simulink model "takeoff_13"  (R2024b)
settings: Solver=ode8  StartTime=0.0  StopTime=300  FixedStep=1e-3  MaxStep=1e-3  RelTol=1e-3
values from neighbouring files (symbols this model uses):
  AircraftData =     [AircraftData.mat]
undefined symbols (not defined in the file or in its folder): alpha_dot_0, alpha_g, CD_g_TO, deg, dt_Hold, gamma_c_deg, h_0, k_alpha_Rot, k_CL_max_Rot, magnitude, rad, s
libraries: aerolibconvert2 x6, slpidlib x3, aerolibatmos2 x1, aerolibasang x1
settings Model: Creator=agode  LastModifiedBy=deluc
settings SolverCC: ZeroCrossAlgorithm=Adaptive
settings DebuggingCC: IgnoredZcDiagnostic=none
settings RTWCC: GPUComputeCapability=3.5

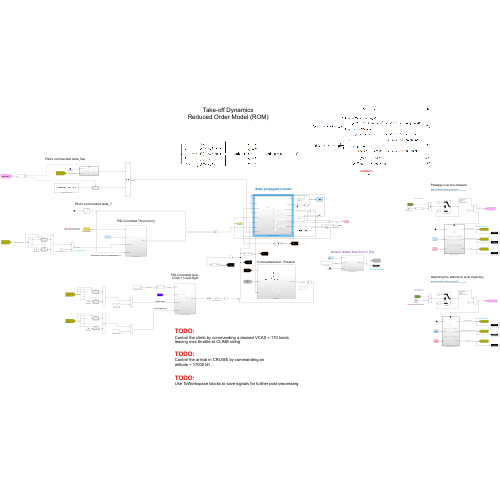
[thumbnail: Simulink's stored preview of the top-level diagram]
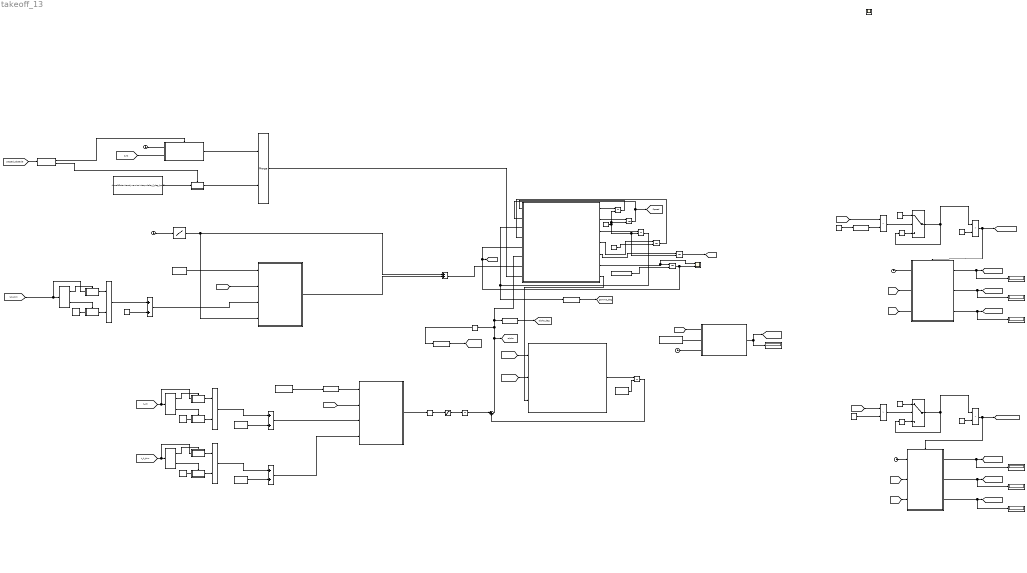
== system takeoff_13 ==
  note: CORRECT:
      | $f_5 = - \dot m_f$
  note: Zero until triggered
  note: Take-off Dynamics
      | Reduced Order Model (ROM)
  note: Detect rotation time from V_Rot
  note: State propagation model
  note: Commanded AoA - Rotation
  note: PID-Controlled AoA - Climb + Level-flight
  note: How to hold the value of a signal?
      | See: https://blogs.mathworks.com/simulink/2014/08/06/how-do-you-hold-the-value-of-a-signal/
  note: Signal may become > X,
      | then < X, then, again > X.
  note: Passage over the obstacle
  note: Zero until triggered
  note: Once this signal
      | becomes = 1,
      | it stays 1
      | (Marcellus Wallace)
  note: Pilot's commanded delta_T
  note: TODO : make this a parameter,
      | taken from performance data
  note: How to hold the value of a signal?
      | See: https://blogs.mathworks.com/simulink/2014/08/06/how-do-you-hold-the-value-of-a-signal/
  note: Zero until triggered
  note: Reaching the altitude to level trajectory
  note: Once this signal
      | becomes = 1,
      | it stays 1
      | (Marcellus Wallace)
  note: Signal may become > X,
      | then < X, then, again > X.
  note: TODO : make this a parameter
  note: PID-Controlled Thrust (trim)
  note: Initial climb
  note: Level trajectory
  note: trim speed: reach a commanded Vc
  note: -1 until triggered
  note: Pilot's commanded delta_flap
  note: TODO:
      | Use ToWorkspace blocks to save signals for further post-processing
  note: TODO:
      | Control the arrival in CRUISE by commanding an altitude = 17000 kft
  note: TODO:
      | Control the climb by commanding a desired VCAS = 170 knots
      | leaving max throttle at CLIMB rating
  1-D Lookup Table : Lookup_n-D  NumberOfTableDimensions=1  BreakpointsForDimension1=[0,2,4,5]  Table=[0, 0.5, 1, 1]  InternalRulePriority=Speed  RndMeth=Simplest
  A/C Reduced Order Dynamics : Subsystem
  Add{,1,3..4} (4 alike) : Sum
  Angle Conversion1 : aerolibconvert2/Angle Conversion  IU=rad  OU=deg
  Angle Conversion2 : aerolibconvert2/Angle Conversion  IU=rad  OU=deg
  Angle Conversion3 : aerolibconvert2/Angle Conversion  IU=deg  OU=rad
  Angular Velocity Conversion3 : aerolibconvert2/Angular Velocity Conversion  IU=rad/s  OU=deg/s
  AoA Control Law in climb : Subsystem
  Clock : Clock
  Clock1 : Clock
  Clock2 : Clock
  Commanded AoA : Subsystem
  Commanded Speed (m/s) : Constant  Value=100
  Commanded gamma (deg) : Constant  Value=gamma_c_deg
  Constant1 : Constant
  Constant2 : Constant  Value=0
  Constant3 : Constant  Value=0
  Constant4 : Constant  Value=alpha_g
  Constant5 : Constant  Value=h_0
  Constant6 : Constant  Value=AircraftData.mass_0
  Constant7 : Constant
  Constant8 : Constant  Value=0
  Derivative : Derivative
  Derivative1 : Derivative
  "Detect S_TO, t_V2, V1" : Subsystem  TreatAsAtomicUnit=on
  "Detect S_TO, t_V2, V2" : Subsystem  TreatAsAtomicUnit=on
  Detect rotation time : Subsystem
  Display{,1..6} (7 alike) : Display
  Flaps at TAKE-OFF position : Constant  Value=AircraftData.Aerodynamics.Interp.delta_f_deg_bp(2)
  Global clock : Clock
  Global clock1 : Clock
  If : If
  If Action Subsystem : Subsystem  TreatAsAtomicUnit=on
  If Action Subsystem1 : Subsystem  TreatAsAtomicUnit=on
  If Action Subsystem2 : Subsystem  TreatAsAtomicUnit=on
  If Action Subsystem3 : Subsystem  TreatAsAtomicUnit=on
  If Action Subsystem4 : Subsystem  TreatAsAtomicUnit=on
  If Action Subsystem5 : Subsystem  TreatAsAtomicUnit=on
  If Action Subsystem6 : Subsystem  TreatAsAtomicUnit=on
  If Action Subsystem7 : Subsystem  TreatAsAtomicUnit=on
  If1 : If
  If2 : If
  If3 : If  IfExpression=u1
  Integrator{,1..6} (7 alike) : Integrator  InitialConditionSource=external
  Integrator7 : Integrator
  Length Conversion : aerolibconvert2/Length Conversion  IU=ft  OU=m
  Memory : Memory
  Memory1 : Memory
  Merge{,1..3} (4 alike) : Merge
  Obstacle height (ft) : Constant  Value=35
  Relational Operator{,1..3} (4 alike) : RelationalOperator  Operator=>  OutDataTypeStr=boolean  RndMeth=Simplest  InputSameDT=off
  Rotation speed : Constant  Value=AircraftData.V_Rot
  Saturation on alpha_dot : Saturate  UpperLimit=12/57.3  LowerLimit=-12/57.3
  Scope : Scope  NumInputPorts=2
  Sum3 : Sum  Inputs=|++
  Switch : Switch  Criteria=u2 > Threshold  SaturateOnIntegerOverflow=off  InputSameDT=off
  Switch1 : Switch  Criteria=u2 > Threshold  SaturateOnIntegerOverflow=off  InputSameDT=off
  Thrust Control Law : Subsystem
  Trim height (m) : Constant  Value=1000
  dummy 0 time : Constant  Value=-11
  level-up decision time (s) : Constant  Value=2
  reaction_time_V2 : Constant  Value=2
  speed-trim decision time (s) : Constant  Value=10
  t_start_climb1 : Constant  Value=1e6
  t_start_climb3 : Constant  Value=1e6
  Angles etc : Scope
  Forces etc : Scope
  tag scope: S_TO=global, S_h_trim=global, Speed=global, alpha=global, alpha_deg=global, alpha_dot_deg_s=global, gamma_deg=global, mass=global, passed_obstacle=global, reached_trim_altitude=global, t_Rot=global, t_V2=global, t_h_trim=global
  wires:
  Commanded AoA/1(AoA_dot (rad/s)) -> Integrator5/1  "alpha_dot (rad/s)"
  Sum3/1 -> Angle Conversion2/1, A/C Reduced Order Dynamics/6(alpha (rad)), Derivative/1, [alpha]
  A/C Reduced Order Dynamics/1(s_dot (m/s)) -> Integrator/1
  A/C Reduced Order Dynamics/2(V_dot (m/s^2)) -> Integrator1/1
  A/C Reduced Order Dynamics/3(gamma_dot (rad/s)) -> Integrator2/1
  A/C Reduced Order Dynamics/4(h_dot (m/s)) -> Integrator3/1
  Integrator1/1 -> A/C Reduced Order Dynamics/2(V (m/s)), [Speed]  "V (m/s)"
  Integrator2/1 -> A/C Reduced Order Dynamics/3(gamma (rad)), Angle Conversion1/1
  Integrator3/1 -> A/C Reduced Order Dynamics/4(h (m))
  Integrator4/1 -> Scope/2, A/C Reduced Order Dynamics/5(mass (kg)), [mass]  "mass (kg)"
  Detect rotation time/1(Rotation time (s)) -> [t_Rot], Display/1
  [Speed] -> Detect rotation time/1(V (m/s))
  Angle Conversion2/1 -> [alpha_deg]  "alpha (deg)"
  Angle Conversion1/1 -> [gamma_deg]  "gamma (deg)"
  Global clock/1 -> Detect rotation time/3(time (s))
  Rotation speed/1 -> Detect rotation time/2(V_Rot (m/s))  "V_Rot (m/s)"
  [t_Rot] -> Commanded AoA/2(t_Rot1)
  [alpha] -> Commanded AoA/1(AoA)
  Integrator5/1 -> Sum3/2
  Commanded gamma (deg)/1 -> Angle Conversion3/1  "gamma_c (deg)"
  Angle Conversion3/1 -> AoA Control Law in climb/1(gamma_c)  "gamma_c"
  [gamma] -> AoA Control Law in climb/2(gamma)
  Angular Velocity Conversion3/1 -> [alpha_dot_deg_s]  "alpha_dot (deg/s)"
  Derivative/1 -> Angular Velocity Conversion3/1
  A/C Reduced Order Dynamics/7(CL) -> Commanded AoA/3(CL)
  A/C Reduced Order Dynamics/6(mass_dot (kg/s)) -> Scope/1, Integrator4/1  "mass_dot (kg/s)"
  A/C Reduced Order Dynamics/5(xE_dot (m/s)) -> Integrator6/1
  Integrator6/1 -> [xE]  "xE (m)"
  [xE] -> "Detect S_TO, t_V2, V2"/3(s (m))
  Relational Operator1/1 -> [passed_obstacle], "Detect S_TO, t_V2, V2"/Trigger
  Constant2/1 -> Relational Operator1/2
  Switch/1 -> Relational Operator1/1, Memory/1
  Relational Operator/1 -> Switch/2
  Memory/1 -> Switch/3
  Constant1/1 -> Switch/1
  [Speed] -> "Detect S_TO, t_V2, V2"/2(V (m/s))
  "Detect S_TO, t_V2, V2"/3(S_ground) -> Display5/1, [S_TO]  "S_TO (m)"
  "Detect S_TO, t_V2, V2"/1(t_LO) -> Display3/1, [t_V2]  "Over-obstacle time (s)"
  "Detect S_TO, t_V2, V2"/2(V_LO) -> Display4/1, [V2_sim]  "Over-obstacle speed sim. (m/s)"
  [h] -> Relational Operator/1
  Clock2/1 -> "Detect S_TO, t_V2, V2"/1(time (s))
  Obstacle height (ft)/1 -> Length Conversion/1
  Length Conversion/1 -> Relational Operator/2
  Integrator/1 -> A/C Reduced Order Dynamics/1(s (m))
  Constant3/1 -> Integrator/2, Integrator1/2, Integrator6/2, Integrator2/2
  Constant5/1 -> Integrator3/2
  Constant6/1 -> Integrator4/2
  Constant4/1 -> Integrator5/2
  Derivative1/1 -> Saturation on alpha_dot/1
  AoA Control Law in climb/1(Delta_alpha) -> Derivative1/1
  Saturation on alpha_dot/1 -> Integrator7/1
  Integrator7/1 -> Sum3/1
  Clock/1 -> 1-D Lookup Table/1
  1-D Lookup Table/1 -> Thrust Control Law/4(Pilot's delta_T), Add/1
  Add/1 -> A/C Reduced Order Dynamics/7(delta_T)
  Thrust Control Law/1(Delta delta_T) -> Add/2
  [Speed] -> Thrust Control Law/2(V)
  Commanded Speed (m/s)/1 -> Thrust Control Law/1(V_c)  "V_c (m/s)"
  reaction_time_V2/1 -> Add1/2
  [t_V2] -> If Action Subsystem/1(In1), If/1
  t_start_climb1/1 -> If Action Subsystem1/1(In1)
  If/1 -> If Action Subsystem/Action
  If/2 -> If Action Subsystem1/Action
  If Action Subsystem/1(Out1) -> Merge/1
  If Action Subsystem1/1(Out1) -> Merge/2
  Merge/1 -> Add1/1
  Add1/1 -> AoA Control Law in climb/3(t_start_climb)
  Constant8/1 -> Relational Operator3/2
  Relational Operator2/1 -> Switch1/2
  [Speed] -> "Detect S_TO, t_V2, V1"/2(V (m/s))
  Memory1/1 -> Switch1/3
  Switch1/1 -> Relational Operator3/1, Memory1/1
  [h] -> Relational Operator2/1
  "Detect S_TO, t_V2, V1"/1(t_h_trim) -> Display1/1, [t_h_trim]  "Level-trajectory time (s)"
  Trim height (m)/1 -> Relational Operator2/2
  Clock1/1 -> "Detect S_TO, t_V2, V1"/1(time (s))
  "Detect S_TO, t_V2, V1"/3(S_h_trim) -> Display6/1, [S_h_trim]  "S_h_trim (m)"
  [xE] -> "Detect S_TO, t_V2, V1"/3(s (m))
  Constant7/1 -> Switch1/1
  "Detect S_TO, t_V2, V1"/2(V_h_trim) -> Display2/1, [V_sim_h_trim]  "Speed at level-trajectory time sim. (m/s)"
  Relational Operator3/1 -> [reached_trim_altitude], "Detect S_TO, t_V2, V1"/Trigger
  If Action Subsystem2/1(Out1) -> Merge1/1
  If Action Subsystem3/1(Out1) -> Merge1/2
  dummy 0 time/1 -> If Action Subsystem3/1(In1)
  If1/1 -> If Action Subsystem2/Action
  If1/2 -> If Action Subsystem3/Action
  [t_h_trim] -> If Action Subsystem4/1(In1), If2/1
  If2/1 -> If Action Subsystem4/Action
  If2/2 -> If Action Subsystem5/Action
  Merge2/1 -> Add3/1
  If Action Subsystem5/1(Out1) -> Merge2/2
  If Action Subsystem4/1(Out1) -> Merge2/1
  level-up decision time (s)/1 -> Add3/2
  t_start_climb3/1 -> If Action Subsystem5/1(In1)
  Add3/1 -> AoA Control Law in climb/4(t_start_level)
  [t_h_trim] -> If Action Subsystem2/1(In1), If1/1  "Level-trajectory trim time (s)"
  speed-trim decision time (s)/1 -> Add4/2
  Merge1/1 -> Add4/1
  Add4/1 -> Thrust Control Law/3(t_start_speed_trim)  "Speed-trim time (s)"
  [passed_obstacle] -> If3/1
  Flaps at TAKE-OFF position/1 -> If Action Subsystem7/1(In1)
  If3/2 -> If Action Subsystem7/Action
  If Action Subsystem7/1(Out1) -> Merge3/2
  Merge3/1 -> A/C Reduced Order Dynamics/8(delta_f (deg))  "delta_f (deg)"
  If3/1 -> If Action Subsystem6/Action
  If Action Subsystem6/1(Out1) -> Merge3/1
  Global clock1/1 -> If Action Subsystem6/1(clock time (s))
  [t_V2] -> If Action Subsystem6/2(t_V2 (s))  "Level-trajectory trim time (s)"

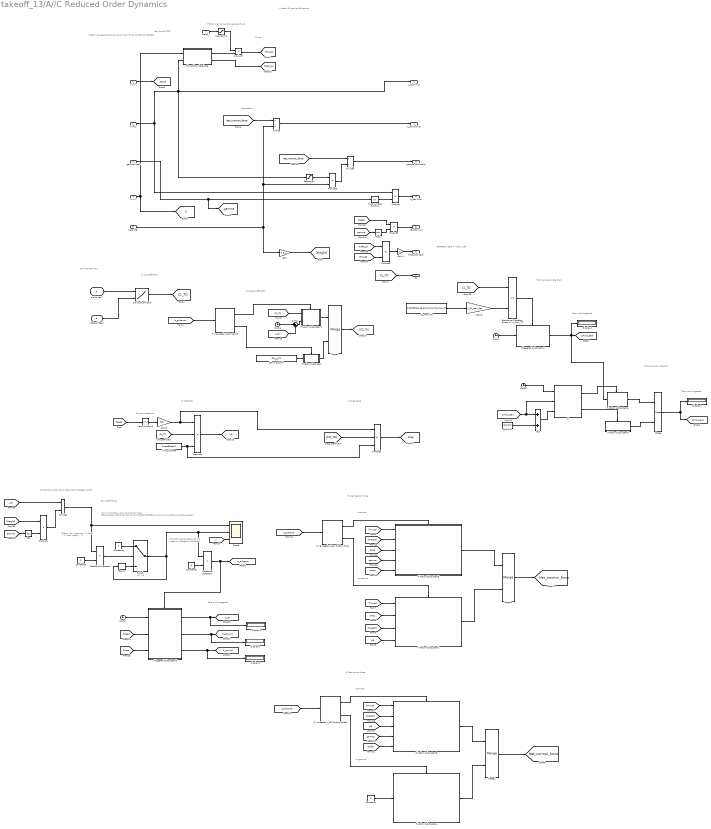
== system takeoff_13/A//C Reduced Order Dynamics ==
  note: TODO: manage the thrust rating, from TO to CLIMB and CRUISE
  note: TODO: plan to handle reverse thrust
  note: on-ground
  note: Commanded
      | AoA
  note: System Dynamics Equations
  note: 3a) Lift-off time
  note: Zero until triggered
  note: 1) Lift coefficient
  note: 3) Lift force
  note: Dinamic pressure
  note: 2) Drag coefficient
  note: 4) Drag force
  note: Max thrust
      | TSFC
  note: 5) Net traction force
  note: Net traction
  note: airborne
  note: 6) Net normal force
  note: on-ground
  note: airborne
  note: Hold AoA grow rate
      | start
  note: Hold AoA grow rate
      | end
  note: Zero until triggered
  note: Zero until triggered
  note: Switching function $S = \frac{L}{W \cos\gamma}$
  note: Once this signal
      | becomes = 1,
      | it stays 1
      | (Marcellus Wallace)
  note: How to hold the value of a signal?
      | See: https://blogs.mathworks.com/simulink/2014/08/06/how-do-you-hold-the-value-of-a-signal/
  note: Signal may become > 1,
      | then < 1, then, again > 1.
  note: Thrust
  note: CORRECT: $f_5 = - \dot m_f$
  s (m) : Inport
  V (m/s) : Inport  Port=2
  gamma (rad) : Inport  Port=3
  h (m) : Inport  Port=4
  mass (kg) : Inport  Port=5
  alpha (rad) : Inport  Port=6
  delta_T : Inport  Port=7  OutDataTypeStr=double
  delta_f (deg) : Inport  Port=8
  2-D Lookup Table : Lookup_n-D  BreakpointsForDimension1=AircraftData.Aerodynamics.Interp.AoA_bp  BreakpointsForDimension2=AircraftData.Aerodynamics.Interp.delta_f_deg_bp  Table=transpose(AircraftData.Aerodynamics.Interp.CL_Interp)  InternalRulePriority=Speed  RndMeth=Simplest
      settings: InputPortMap=u0,u1
  Add : Sum
  CD on ground : Constant  Value=CD_g_TO
  CL_max_TO : Constant  Value=AircraftData.Aerodynamics.CL_max_TO
  Clock{,1..3} (4 alike) : Clock
  Constant1 : Constant  Value=0
  Constant3 : Constant
  Constant4 : Constant
  Constant5 : Constant  Value=0
  Cos : Trigonometry  Operator=cos
  Cos1 : Trigonometry  Operator=cos
  Display{1..5} (5 alike) : Display
  Divide : Product  Inputs=*/
  Divide1 : Product  Inputs=*/
  Divide2 : Product  Inputs=*/
  Gain : Gain  Gain=9.81
  Gain1 : Gain  Gain=-1
  Gain3 : Gain  Gain=k_CL_max_Rot
  Gain5 : Gain  Gain=0.5
  If : If  NumInputs=3  IfExpression=u2 > 0 & u1 > u3
  If Action Subsystem : Subsystem  TreatAsAtomicUnit=on
  If Action Subsystem1 : Subsystem  TreatAsAtomicUnit=on
  If Action Subsystem2 : Subsystem  TreatAsAtomicUnit=on
  If Action Subsystem3 : Subsystem  TreatAsAtomicUnit=on
  If Action Subsystem4 : Subsystem  TreatAsAtomicUnit=on
  If Action Subsystem5 : Subsystem  TreatAsAtomicUnit=on
  If Action Subsystem6 : Subsystem  TreatAsAtomicUnit=on
  If Action Subsystem7 : Subsystem  TreatAsAtomicUnit=on
  If V exceeds V_LO: CD_TO : If  IfExpression=u1
  If V exceeds V_LO: Friction force : If  IfExpression=u1
  If V exceeds V_LO: Friction force1 : If  IfExpression=u1
  Math Function1 : Math  Operator=square
  Memory : Memory
  Merge{,1..3} (4 alike) : Merge
  Product{,3..7} (6 alike) : Product
  Product1 : Product  Inputs=3
  Product2 : Product  Inputs=3
  Relational Operator : RelationalOperator  Operator=>  OutDataTypeStr=boolean  RndMeth=Simplest  InputSameDT=off
  Relational Operator. Event: CL exceed k*CL_max_TO : RelationalOperator  OutDataTypeStr=boolean  RndMeth=Simplest  InputSameDT=off
  Relational Operator1 : RelationalOperator  Operator=>  OutDataTypeStr=boolean  RndMeth=Simplest  InputSameDT=off
  Saturation : Saturate  UpperLimit=1e8  LowerLimit=1e-9
  Saturation1 : Saturate  UpperLimit=1  LowerLimit=0
  Scope : Scope  NumInputPorts=3
  Sum2 : Sum  Inputs=|+-
  Switch : Switch  Criteria=u2 > Threshold  SaturateOnIntegerOverflow=off  InputSameDT=off
  Thrust from database : Subsystem
  Triggered Subsystem1 : Subsystem  TreatAsAtomicUnit=on
  Triggered Subsystem2 : Subsystem  TreatAsAtomicUnit=on
  Trigonometric Function : Trigonometry
  Wing Surface : Constant  Value=AircraftData.S
  dt_Hold1 : Constant  Value=dt_Hold
  s_dot (m/s) : Outport
  V_dot (m/s^2) : Outport  Port=2
  gamma_dot (rad/s) : Outport  Port=3
  h_dot (m/s) : Outport  Port=4
  xE_dot (m/s) : Outport  Port=5
  mass_dot (kg/s) : Outport  Port=6
  CL : Outport  Port=7
  tag scope: CL_TO=global, Drag=global, Lift=global, Net_normal_force=global, Net_traction_force=global, S_ground=global, Space=global, gamma=global, h=global, is_airborne=global, t_Hold_end=global, t_Hold_start=global, t_LO=global
  wires:
  V (m/s)/1 -> Product/1, Saturation/1, Thrust from database/2(Speed (m/s)), s_dot (m/s)/1  "V (m/s)"
  s (m)/1 -> [Space]
  mass (kg)/1 -> Gain/1, Divide/2, Product3/2  "mass (kg)"
  gamma (rad)/1 -> Trigonometric Function/1, [gamma]  "gamma (rad)"
  Trigonometric Function/1 -> Product/2
  Product/1 -> h_dot (m/s)/1
  Triggered Subsystem2/2(V_LO) -> Display4/1, [V_LO_sim]  "Lift-off speed sim. (m/s)"
  Clock2/1 -> Triggered Subsystem2/1(time (s))
  Triggered Subsystem2/1(t_LO) -> [t_LO], Display3/1  "Lift-off time (s)"
  [Speed] -> Triggered Subsystem2/2(V (m/s))
  h (m)/1 -> [h], Thrust from database/1(Altitude (m))  "h (m)"
  [Net_traction_force] -> Divide/1  "Net traction (N)"
  Divide/1 -> V_dot (m/s^2)/1
  2-D Lookup Table/1 -> [CL_TO]  "CL"
  alpha (rad)/1 -> 2-D Lookup Table/1
  Gain5/1 -> Product2/1, Product1/1  "Dynamic pressure (N)"
  Math Function1/1 -> Gain5/1
  Product1/1 -> [Lift]  "Lift (N)"
  [Speed] -> Math Function1/1
  If V exceeds V_LO: CD_TO/1 -> If Action Subsystem1/Action
  [is_airborne] -> If V exceeds V_LO: CD_TO/1  "is_above_V_LO"
  CD on ground/1 -> If Action Subsystem/1(In1)
  Merge2/1 -> [CD_TO]
  If Action Subsystem1/1(CD_TO) -> Merge2/1
  Sum2/1 -> If Action Subsystem1/2(t - t_LO)
  If Action Subsystem/1(Out1) -> Merge2/2
  If V exceeds V_LO: CD_TO/2 -> If Action Subsystem/Action
  [t_LO] -> Sum2/2
  Clock1/1 -> Sum2/1
  [CL_TO] -> If Action Subsystem1/1(CL_TO)
  Product2/1 -> [Drag]  "Drag (N)"
  [CL_TO] -> Product1/2
  Wing Surface/1 -> Product2/3, Product1/3
  [CD_TO] -> Product2/2
  [Drag] -> If Action Subsystem2/2(Drag)
  If Action Subsystem2/1(Net traction force on-ground) -> Merge3/2
  [is_airborne] -> If V exceeds V_LO: Friction force/1  "is_above_V_LO"
  If V exceeds V_LO: Friction force/1 -> If Action Subsystem3/Action
  If Action Subsystem3/1(Net traction force airborne) -> Merge3/1  "Net traction force airborne (N)"
  If V exceeds V_LO: Friction force/2 -> If Action Subsystem2/Action
  Gain/1 -> [Weight]  "Weight (N)"
  Merge3/1 -> [Net_traction_force]  "Net traction force (N)"
  [Lift] -> If Action Subsystem2/4(Lift)
  [Weight] -> If Action Subsystem2/3(Weight)
  [Thrust] -> If Action Subsystem2/1(Thrust)
  [Thrust] -> If Action Subsystem3/1(Thrust)
  [Weight] -> If Action Subsystem3/2(Weight)
  [Drag] -> If Action Subsystem3/3(Drag)
  [Thrust] -> If Action Subsystem5/1(Thrust)
  [Lift] -> If Action Subsystem5/3(Lift)
  [gamma] -> If Action Subsystem5/4(gamma)
  If V exceeds V_LO: Friction force1/2 -> If Action Subsystem4/Action
  If Action Subsystem5/1(Net normal force airborne) -> Merge1/1
  [is_airborne] -> If V exceeds V_LO: Friction force1/1  "is_above_V_LO"
  If Action Subsystem4/1(Net normal force on-ground) -> Merge1/2
  Merge1/1 -> [Net_normal_force]  "Net traction force (N)"
  If V exceeds V_LO: Friction force1/1 -> If Action Subsystem5/Action
  [Weight] -> If Action Subsystem5/2(Weight)
  Constant1/1 -> If Action Subsystem4/1(in1)
  [alpha] -> If Action Subsystem3/5(AoA)
  [gamma] -> If Action Subsystem3/4(gamma)
  [alpha] -> If Action Subsystem5/5(AoA)
  [Net_normal_force] -> Divide1/1  "Net norm. force (N)"
  Product3/1 -> Divide1/2
  Triggered Subsystem1/1(t_Hold_start) -> If Action Subsystem6/1(t_Hold_start), Display2/1, [t_Hold_start]  "Hold time start (s)"
  Clock/1 -> Triggered Subsystem1/1(time (s))
  Relational Operator. Event: CL exceed k*CL_max_TO/1 -> Triggered Subsystem1/Trigger
  CL_max_TO/1 -> Gain3/1  "CL_max"
  Divide1/1 -> gamma_dot (rad/s)/1
  Saturation/1 -> Product3/1
  [CL_TO] -> Relational Operator. Event: CL exceed k*CL_max_TO/1
  Gain3/1 -> Relational Operator. Event: CL exceed k*CL_max_TO/2  "CL_Hold_start"
  [Lift] -> Divide2/1
  [Weight] -> Product4/1
  Cos/1 -> Product4/2
  [gamma] -> Cos/1
  Product4/1 -> Divide2/2
  Divide2/1 -> Relational Operator/1, Scope/1  "Switching func"
  Merge/1 -> [t_Hold_end], Display1/1  "Hold time end (s)"
  Clock3/1 -> If/1
  [t_Hold_start] -> If/2, Add/1
  dt_Hold1/1 -> Add/2
  If/1 -> If Action Subsystem6/Action
  If Action Subsystem6/1(Out1) -> Merge/1
  If Action Subsystem7/1(Zero (s)) -> Merge/2
  If/2 -> If Action Subsystem7/Action
  Add/1 -> If/3
  Constant4/1 -> Switch/1
  Constant3/1 -> Relational Operator/2
  Switch/1 -> Relational Operator1/1, Scope/2, Memory/1
  Relational Operator/1 -> Switch/2
  Memory/1 -> Switch/3
  Constant5/1 -> Relational Operator1/2
  Relational Operator1/1 -> Triggered Subsystem2/Trigger, [is_airborne]
  [h] -> Scope/3
  [Space] -> Triggered Subsystem2/3(s (m))
  Triggered Subsystem2/3(S_ground) -> Display5/1, [S_ground]  "S_ground (m)"
  [CL_TO] -> CL/1
  [Speed] -> Product5/1
  [gamma] -> Cos1/1
  Cos1/1 -> Product5/2
  Product5/1 -> xE_dot (m/s)/1
  [TSFC_SI] -> Product6/1
  [Thrust] -> Product6/2
  Product6/1 -> Gain1/1
  Gain1/1 -> mass_dot (kg/s)/1
  Product7/1 -> [Thrust]  "Thrust (N)"
  Thrust from database/1(Max Thrust (N)) -> Product7/2  "Thrust_max (N)"
  delta_T/1 -> Saturation1/1
  Saturation1/1 -> Product7/1
  Thrust from database/2(TSFC kg/(N*s)) -> [TSFC_SI]
  delta_f (deg)/1 -> 2-D Lookup Table/2

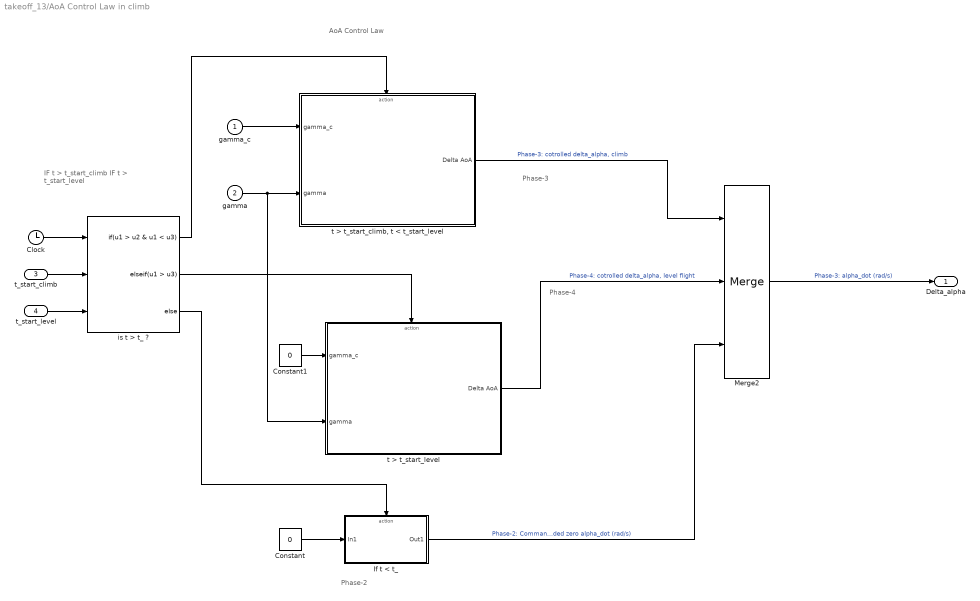
== system takeoff_13/AoA Control Law in climb ==
  note: Phase-3
  note: IF t > t_start_climb
      | IF t > t_start_level
  note: Phase-2
  note: AoA Control Law
  note: Phase-4
  gamma_c : Inport
  gamma : Inport  Port=2
  t_start_climb : Inport  Port=3
  t_start_level : Inport  Port=4
  Clock : Clock
  Constant : Constant  Value=0
  Constant1 : Constant  Value=0
  If t < t_ : Subsystem  TreatAsAtomicUnit=on
  Merge2 : Merge  Inputs=3
  is t > t_ ? : If  NumInputs=3  IfExpression=u1 > u2 & u1 < u3  ElseIfExpressions=u1 > u3
  "t > t_start_climb, t < t_start_level" : Subsystem  TreatAsAtomicUnit=on
  t > t_start_level : Subsystem  TreatAsAtomicUnit=on
  Delta_alpha : Outport
  wires:
  gamma_c/1 -> "t > t_start_climb, t < t_start_level"/1(gamma_c)
  gamma/1 -> t > t_start_level/2(gamma), "t > t_start_climb, t < t_start_level"/2(gamma)
  If t < t_/1(Out1) -> Merge2/3  "Phase-2: Commanded zero alpha_dot (rad/s)"
  t_start_climb/1 -> is t > t_ ?/2
  "t > t_start_climb, t < t_start_level"/1(Delta AoA) -> Merge2/1  "Phase-3: cotrolled delta_alpha, climb"
  is t > t_ ?/1 -> "t > t_start_climb, t < t_start_level"/Action
  is t > t_ ?/3 -> If t < t_/Action
  Constant/1 -> If t < t_/1(In1)
  Merge2/1 -> Delta_alpha/1  "Phase-3: alpha_dot (rad/s)"
  Clock/1 -> is t > t_ ?/1
  t_start_level/1 -> is t > t_ ?/3
  is t > t_ ?/2 -> t > t_start_level/Action
  Constant1/1 -> t > t_start_level/1(gamma_c)
  t > t_start_level/1(Delta AoA) -> Merge2/2  "Phase-4: cotrolled delta_alpha, level flight"

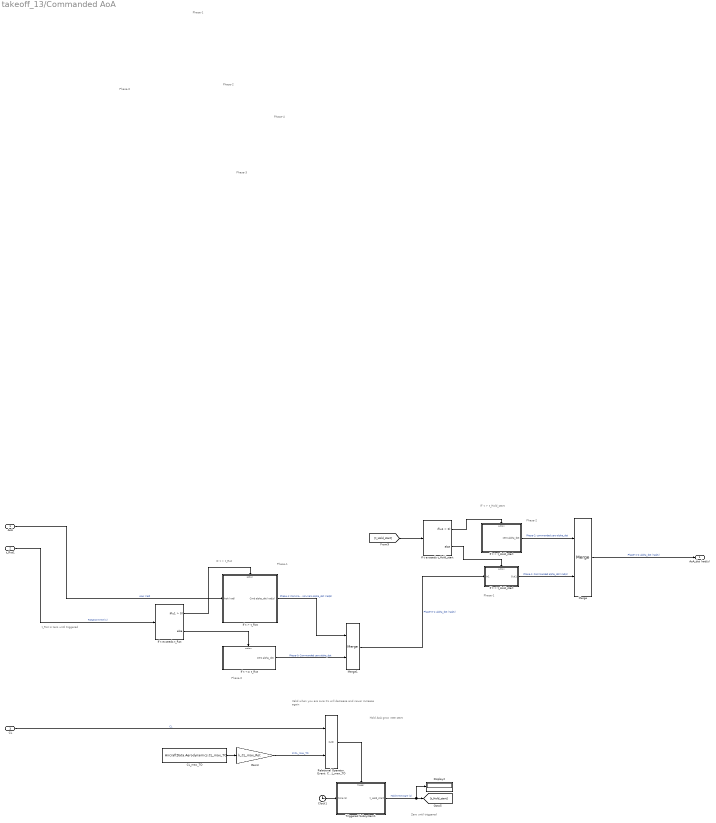
== system takeoff_13/Commanded AoA ==
  note: IF t > t_Rot
  note: t_Rot is zero until triggered
  note: Hold AoA grow rate
      | start
  note: Zero until triggered
  note: IF t > t_Hold_start
  note: Valid when you are sure CL will decrease and never increase again
  note: Phase-0
  note: Phase-1
  note: Phase-2
  note: Phase-3
  note: Phase-4
  note: Phase-0
  note: Phase-1
  note: Phase-1
  note: Phase-2
  AoA : Inport
  t_Rot1 : Inport  Port=2
  CL : Inport  Port=3
  CL_max_TO : Constant  Value=AircraftData.Aerodynamics.CL_max_TO
  Clock1 : Clock
  Display2 : Display
  Gain3 : Gain  Gain=k_CL_max_Rot
  If t < t_Hold_start : Subsystem  TreatAsAtomicUnit=on
  If t <= t_Rot : Subsystem  TreatAsAtomicUnit=on
  If t > t_Hold_start : Subsystem  TreatAsAtomicUnit=on
  If t > t_Rot : Subsystem  TreatAsAtomicUnit=on
  If t exceeds t_Hold_start : If
  If t exceeds t_Rot : If
  Merge : Merge
  Merge1 : Merge
  Relational Operator. Event: CL exceed k*CL_max_TO : RelationalOperator  OutDataTypeStr=boolean  RndMeth=Simplest  InputSameDT=off
  Triggered Subsystem1 : Subsystem  TreatAsAtomicUnit=on
  AoA_dot (rad/s) : Outport
  wires:
  If t > t_Rot/1(Cmd alpha_dot (rad/s)) -> Merge1/1  "Phase-1: Commanded non-zero alpha_dot (rad/s)"
  t_Rot1/1 -> If t exceeds t_Rot/1  "Rotation time (s)"
  If t exceeds t_Rot/2 -> If t <= t_Rot/Action
  If t <= t_Rot/1(zero alpha_dot) -> Merge1/2  "Phase-0: Commanded zero alpha_dot"
  AoA/1 -> If t > t_Rot/1(AoA (rad))  "AoA (rad)"
  If t exceeds t_Rot/1 -> If t > t_Rot/Action
  Triggered Subsystem1/1(t_Hold_start) -> Display2/1, [t_Hold_start]  "Hold time start (s)"
  Clock1/1 -> Triggered Subsystem1/1(time (s))
  Relational Operator. Event: CL exceed k*CL_max_TO/1 -> Triggered Subsystem1/Trigger
  CL_max_TO/1 -> Gain3/1
  Gain3/1 -> Relational Operator. Event: CL exceed k*CL_max_TO/2  "k*CL_max_TO"
  CL/1 -> Relational Operator. Event: CL exceed k*CL_max_TO/1  "CL"
  If t < t_Hold_start/1(Out1) -> Merge/2  "Phase-1: Commanded alpha_dot (rad/s)"
  If t exceeds t_Hold_start/1 -> If t > t_Hold_start/Action
  Merge1/1 -> If t < t_Hold_start/1(In1)  "Phase-0-1: alpha_dot (rad/s)"
  If t exceeds t_Hold_start/2 -> If t < t_Hold_start/Action
  If t > t_Hold_start/1(zero alpha_dot) -> Merge/1  "Phase-2: commanded zero alpha_dot"
  [t_Hold_start] -> If t exceeds t_Hold_start/1
  Merge/1 -> AoA_dot (rad/s)/1  "Phase-1-2: alpha_dot (rad/s)"

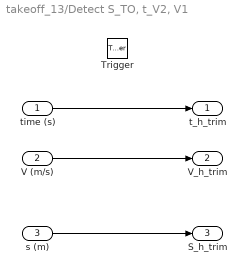
== system takeoff_13/Detect S_TO, t_V2, V1 ==
  time (s) : Inport
  V (m/s) : Inport  Port=2
  s (m) : Inport  Port=3
  Trigger : TriggerPort  VariantControl=(inherit)
  t_h_trim : Outport
  V_h_trim : Outport  Port=2
  S_h_trim : Outport  Port=3
  wires:
  time (s)/1 -> t_h_trim/1
  V (m/s)/1 -> V_h_trim/1
  s (m)/1 -> S_h_trim/1

== system takeoff_13/Detect S_TO, t_V2, V2 ==
  time (s) : Inport
  V (m/s) : Inport  Port=2
  s (m) : Inport  Port=3
  Trigger : TriggerPort  VariantControl=(inherit)
  t_LO : Outport
  V_LO : Outport  Port=2
  S_ground : Outport  Port=3
  wires:
  time (s)/1 -> t_LO/1
  V (m/s)/1 -> V_LO/1
  s (m)/1 -> S_ground/1

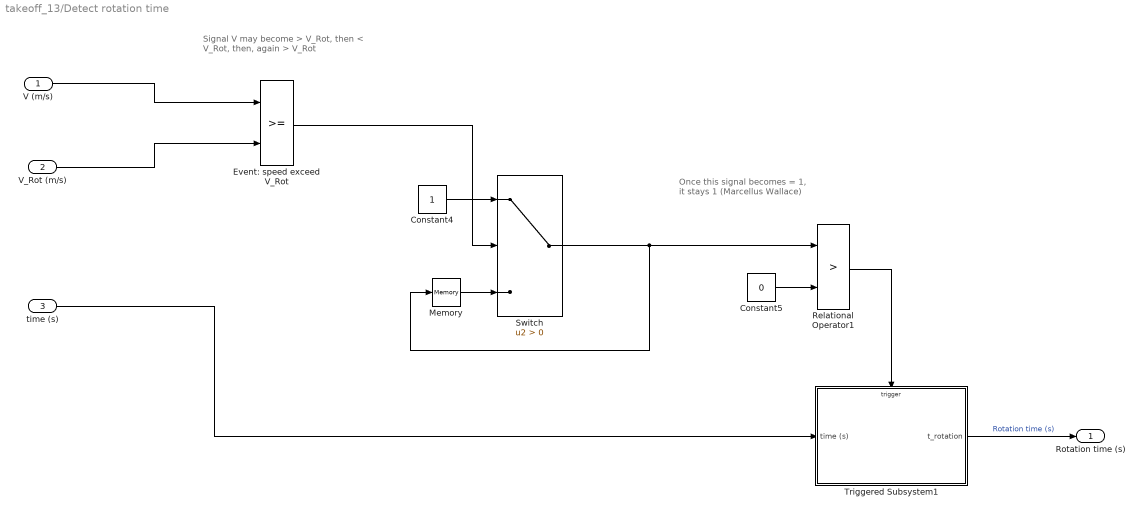
== system takeoff_13/Detect rotation time ==
  note: Signal V may become > V_Rot,
      | then < V_Rot, then, again > V_Rot
  note: Once this signal
      | becomes = 1,
      | it stays 1
      | (Marcellus Wallace)
  V (m/s) : Inport
  V_Rot (m/s) : Inport  Port=2
  time (s) : Inport  Port=3
  Constant4 : Constant
  Constant5 : Constant  Value=0
  Event: speed exceed V_Rot : RelationalOperator  OutDataTypeStr=boolean  RndMeth=Simplest  InputSameDT=off
  Memory : Memory
  Relational Operator1 : RelationalOperator  Operator=>  OutDataTypeStr=boolean  RndMeth=Simplest  InputSameDT=off
  Switch : Switch  Criteria=u2 > Threshold  SaturateOnIntegerOverflow=off  InputSameDT=off
  Triggered Subsystem1 : Subsystem  TreatAsAtomicUnit=on
  Rotation time (s) : Outport
  wires:
  V (m/s)/1 -> Event: speed exceed V_Rot/1
  time (s)/1 -> Triggered Subsystem1/1(time (s))
  Event: speed exceed V_Rot/1 -> Switch/2
  Switch/1 -> Relational Operator1/1, Memory/1
  Memory/1 -> Switch/3
  V_Rot (m/s)/1 -> Event: speed exceed V_Rot/2
  Constant4/1 -> Switch/1
  Constant5/1 -> Relational Operator1/2
  Relational Operator1/1 -> Triggered Subsystem1/Trigger
  Triggered Subsystem1/1(t_rotation) -> Rotation time (s)/1  "Rotation time (s)"

== system takeoff_13/If Action Subsystem ==
  In1 : Inport
  Action Port : ActionPort  ActionPortLabel=if(u1 > 0)
  Out1 : Outport
  wires:
  In1/1 -> Out1/1

== system takeoff_13/If Action Subsystem1 ==
  In1 : Inport
  Action Port : ActionPort  ActionPortLabel=else
  Out1 : Outport
  wires:
  In1/1 -> Out1/1

== system takeoff_13/If Action Subsystem2 ==
  In1 : Inport
  Action Port : ActionPort  ActionPortLabel=if(u1 > 0)
  Out1 : Outport
  wires:
  In1/1 -> Out1/1

== system takeoff_13/If Action Subsystem3 ==
  In1 : Inport
  Action Port : ActionPort  ActionPortLabel=else
  Out1 : Outport
  wires:
  In1/1 -> Out1/1

== system takeoff_13/If Action Subsystem4 ==
  In1 : Inport
  Action Port : ActionPort  ActionPortLabel=if(u1 > 0)
  Out1 : Outport
  wires:
  In1/1 -> Out1/1

== system takeoff_13/If Action Subsystem5 ==
  In1 : Inport
  Action Port : ActionPort  ActionPortLabel=else
  Out1 : Outport
  wires:
  In1/1 -> Out1/1

== system takeoff_13/If Action Subsystem6 ==
  clock time (s) : Inport
  t_V2 (s) : Inport  Port=2
  Action Port : ActionPort  ActionPortLabel=if(u1)
  1-D Lookup Table: delay then ramp down to CLEAN CL(alpha) : Lookup_n-D  NumberOfTableDimensions=1  BreakpointsForDimension1=[0, 5 + 1.5*[0:5,6]]  Table="AircraftData.Aerodynamics.Interp.delta_f_deg_bp(2)*[1,(1 -  [tanh([0:5]),1])]"  InternalRulePriority=Speed  RndMeth=Simplest
  Add : Sum  Inputs=+-
  Scope : Scope
  Out1 : Outport
  wires:
  clock time (s)/1 -> Add/1
  t_V2 (s)/1 -> Add/2
  Add/1 -> 1-D Lookup Table: delay then ramp down to CLEAN CL(alpha)/1
  1-D Lookup Table: delay then ramp down to CLEAN CL(alpha)/1 -> Scope/1, Out1/1

== system takeoff_13/If Action Subsystem7 ==
  In1 : Inport
  Action Port : ActionPort  ActionPortLabel=else
  Out1 : Outport
  wires:
  In1/1 -> Out1/1

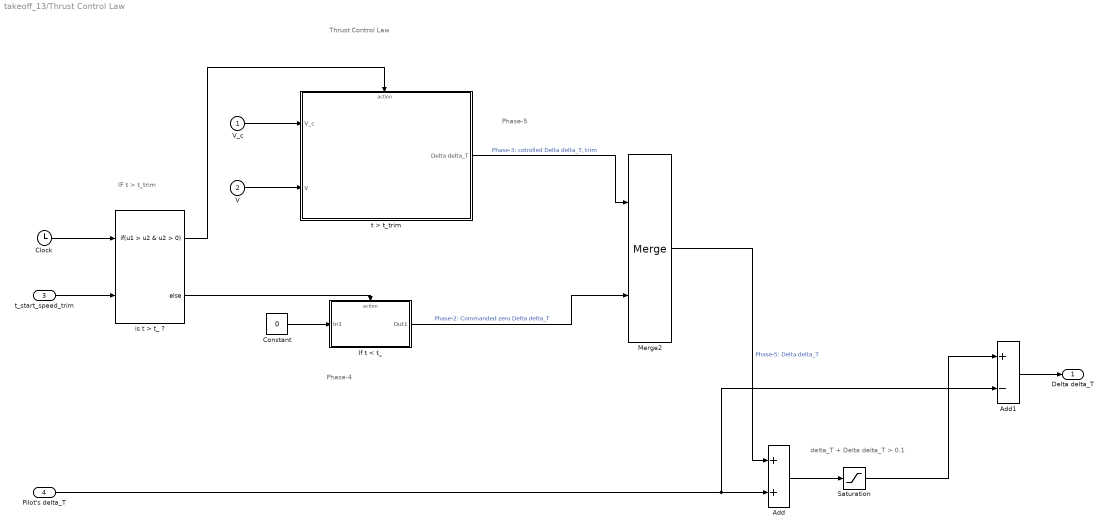
== system takeoff_13/Thrust Control Law ==
  note: delta_T + Delta delta_T > 0.1
  note: Phase-5
  note: IF t > t_trim
  note: Phase-4
  note: Thrust Control Law
  V_c : Inport
  V : Inport  Port=2
  t_start_speed_trim : Inport  Port=3
  Pilot's delta_T : Inport  Port=4
  Add : Sum
  Add1 : Sum  Inputs=+-
  Clock : Clock
  Constant : Constant  Value=0
  If t < t_ : Subsystem  TreatAsAtomicUnit=on
  Merge2 : Merge
  Saturation : Saturate  UpperLimit=1  LowerLimit=0.1
  is t > t_ ? : If  NumInputs=2  IfExpression=u1 > u2 & u2 > 0
  t > t_trim : Subsystem  TreatAsAtomicUnit=on
  Delta delta_T : Outport
  wires:
  V_c/1 -> t > t_trim/1(V_c)
  V/1 -> t > t_trim/2(V)
  If t < t_/1(Out1) -> Merge2/2  "Phase-2: Commanded zero Delta delta_T"
  t_start_speed_trim/1 -> is t > t_ ?/2
  t > t_trim/1(Delta delta_T) -> Merge2/1  "Phase-3: cotrolled Delta delta_T, trim"
  is t > t_ ?/1 -> t > t_trim/Action
  is t > t_ ?/2 -> If t < t_/Action
  Constant/1 -> If t < t_/1(In1)
  Merge2/1 -> Add/1  "Phase-5: Delta delta_T"
  Clock/1 -> is t > t_ ?/1
  Pilot's delta_T/1 -> Add1/2, Add/2
  Add/1 -> Saturation/1
  Saturation/1 -> Add1/1
  Add1/1 -> Delta delta_T/1

== system takeoff_13/A//C Reduced Order Dynamics/If Action Subsystem ==
  In1 : Inport
  Action Port : ActionPort  ActionPortLabel=else
  Out1 : Outport
  wires:
  In1/1 -> Out1/1

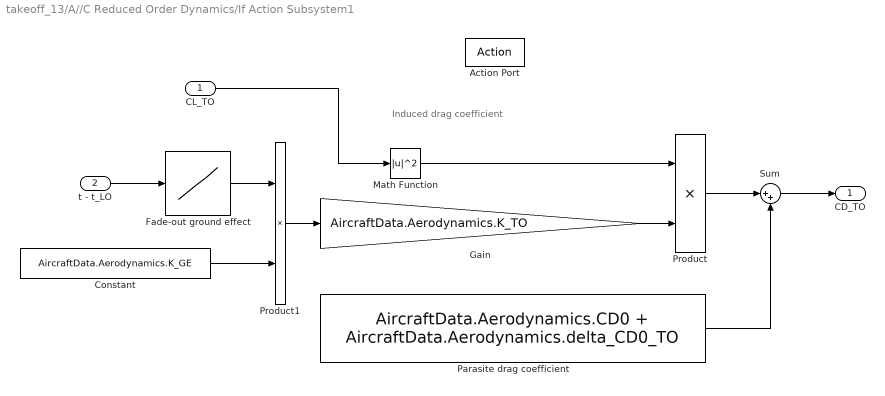
== system takeoff_13/A//C Reduced Order Dynamics/If Action Subsystem1 ==
  note: Induced drag coefficient
  CL_TO : Inport
  t - t_LO : Inport  Port=2
  Action Port : ActionPort  ActionPortLabel=if(u1)
  Constant : Constant  Value=AircraftData.Aerodynamics.K_GE
  Fade-out ground effect : Lookup_n-D  NumberOfTableDimensions=1  BreakpointsForDimension1=(1/6.0)*[0:6]  Table=1 - tanh([0:6])  InternalRulePriority=Speed  RndMeth=Simplest
  Gain : Gain  Gain=AircraftData.Aerodynamics.K_TO
  Math Function : Math  Operator=magnitude^2
  Parasite drag coefficient : Constant  Value=AircraftData.Aerodynamics.CD0 + AircraftData.Aerodynamics.delta_CD0_TO
  Product : Product
  Product1 : Product
  Sum : Sum  Inputs=|++
  CD_TO : Outport
  wires:
  Gain/1 -> Product/2
  Math Function/1 -> Product/1
  Product/1 -> Sum/1
  CL_TO/1 -> Math Function/1
  Parasite drag coefficient/1 -> Sum/2
  Sum/1 -> CD_TO/1
  Fade-out ground effect/1 -> Product1/1
  Constant/1 -> Product1/2
  Product1/1 -> Gain/1
  t - t_LO/1 -> Fade-out ground effect/1

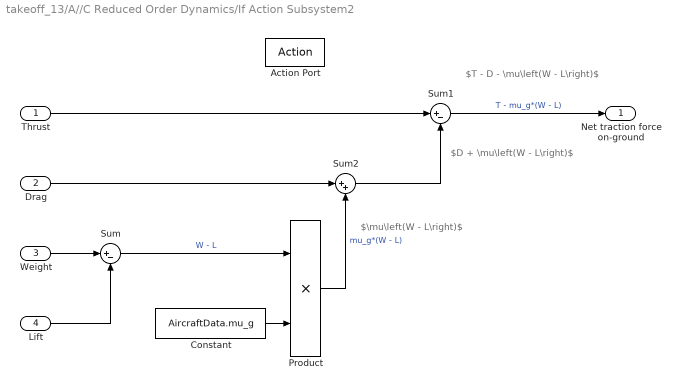
== system takeoff_13/A//C Reduced Order Dynamics/If Action Subsystem2 ==
  note: $T - D - \mu\left(W - L\right)$
  note: $D + \mu\left(W - L\right)$
  note: $\mu\left(W - L\right)$
  Thrust : Inport
  Drag : Inport  Port=2
  Weight : Inport  Port=3
  Lift : Inport  Port=4
  Action Port : ActionPort  ActionPortLabel=else
  Constant : Constant  Value=AircraftData.mu_g
  Product : Product
  Sum : Sum  Inputs=|+-
  Sum1 : Sum  Inputs=|+-
  Sum2 : Sum  Inputs=|++
  Net traction force on-ground : Outport
  wires:
  Constant/1 -> Product/2
  Sum/1 -> Product/1  "W - L"
  Thrust/1 -> Sum1/1
  Sum1/1 -> Net traction force on-ground/1  "T - mu_g*(W - L)"
  Weight/1 -> Sum/1
  Lift/1 -> Sum/2
  Drag/1 -> Sum2/1
  Product/1 -> Sum2/2  "mu_g*(W - L)"
  Sum2/1 -> Sum1/2

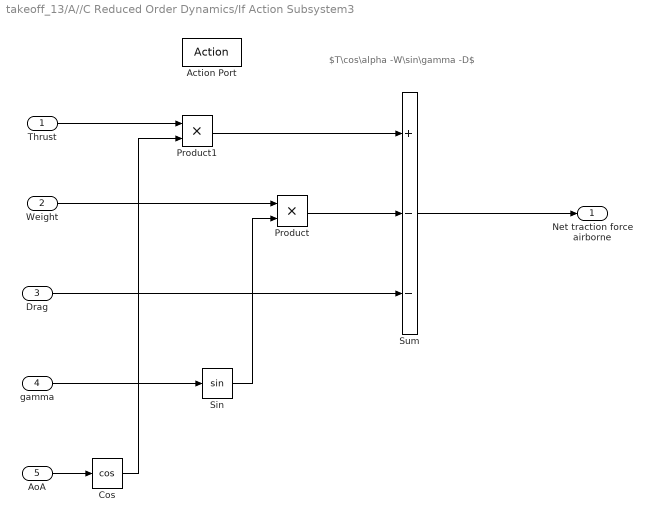
== system takeoff_13/A//C Reduced Order Dynamics/If Action Subsystem3 ==
  note: $T\cos\alpha -W\sin\gamma -D$
  Thrust : Inport
  Weight : Inport  Port=2
  Drag : Inport  Port=3
  gamma : Inport  Port=4
  AoA : Inport  Port=5
  Action Port : ActionPort  ActionPortLabel=if(u1)
  Cos : Trigonometry  Operator=cos
  Product : Product
  Product1 : Product
  Sin : Trigonometry
  Sum : Sum  Inputs=+--
  Net traction force airborne : Outport
  wires:
  AoA/1 -> Cos/1
  gamma/1 -> Sin/1
  Weight/1 -> Product/1
  Sin/1 -> Product/2
  Thrust/1 -> Product1/1
  Cos/1 -> Product1/2
  Product1/1 -> Sum/1
  Product/1 -> Sum/2
  Drag/1 -> Sum/3
  Sum/1 -> Net traction force airborne/1

== system takeoff_13/A//C Reduced Order Dynamics/If Action Subsystem4 ==
  in1 : Inport
  Action Port : ActionPort  ActionPortLabel=else
  Net normal force on-ground : Outport
  wires:
  in1/1 -> Net normal force on-ground/1

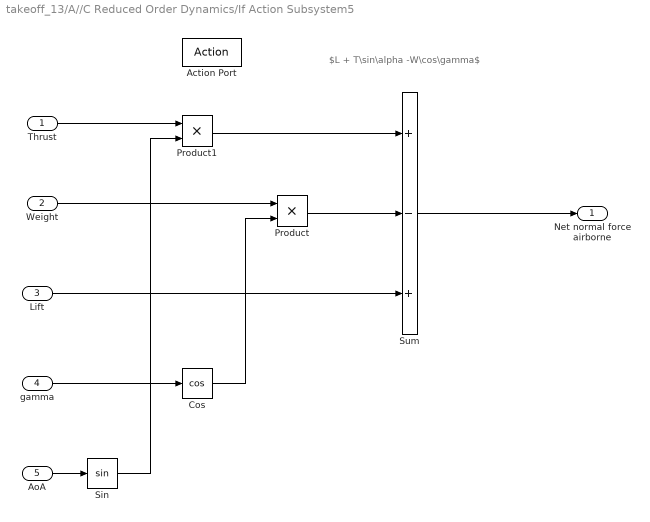
== system takeoff_13/A//C Reduced Order Dynamics/If Action Subsystem5 ==
  note: $L + T\sin\alpha -W\cos\gamma$
  Thrust : Inport
  Weight : Inport  Port=2
  Lift : Inport  Port=3
  gamma : Inport  Port=4
  AoA : Inport  Port=5
  Action Port : ActionPort  ActionPortLabel=if(u1)
  Cos : Trigonometry  Operator=cos
  Product : Product
  Product1 : Product
  Sin : Trigonometry
  Sum : Sum  Inputs=+-+
  Net normal force airborne : Outport
  wires:
  Weight/1 -> Product/1
  Thrust/1 -> Product1/1
  Product1/1 -> Sum/1
  Product/1 -> Sum/2
  Lift/1 -> Sum/3
  Sum/1 -> Net normal force airborne/1
  AoA/1 -> Sin/1
  Sin/1 -> Product1/2
  gamma/1 -> Cos/1
  Cos/1 -> Product/2

== system takeoff_13/A//C Reduced Order Dynamics/If Action Subsystem6 ==
  t_Hold_start : Inport
  Action Port : ActionPort  ActionPortLabel=if(u2 > 0 & u1 > u3)
  Add : Sum
  dt_Hold1 : Constant  Value=dt_Hold
  Out1 : Outport
  wires:
  t_Hold_start/1 -> Add/1
  dt_Hold1/1 -> Add/2
  Add/1 -> Out1/1

== system takeoff_13/A//C Reduced Order Dynamics/If Action Subsystem7 ==
  Action Port : ActionPort  ActionPortLabel=else
  zero : Constant  Value=0
  Zero (s) : Outport
  wires:
  zero/1 -> Zero (s)/1

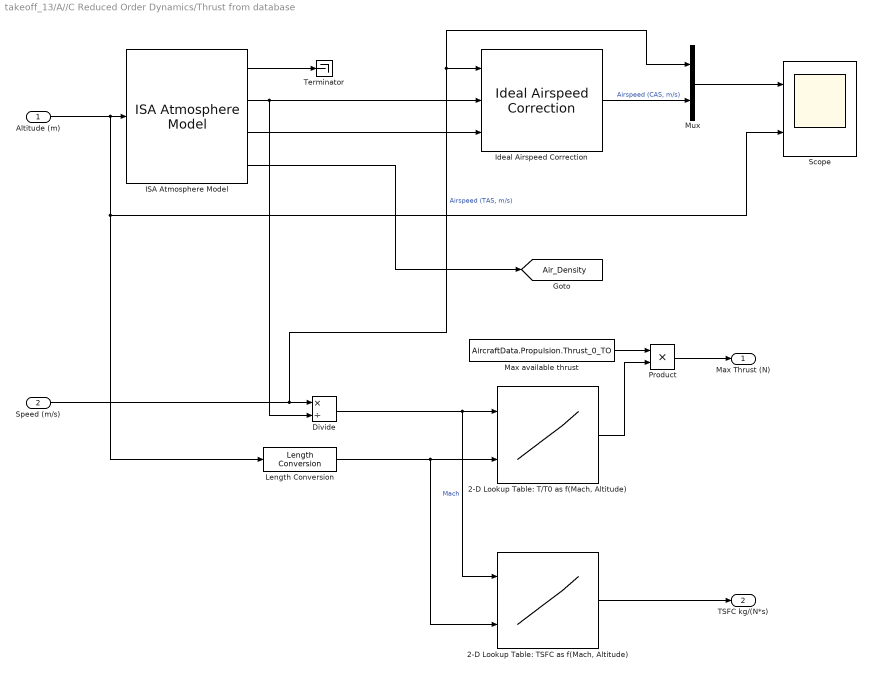
== system takeoff_13/A//C Reduced Order Dynamics/Thrust from database ==
  Altitude (m) : Inport
  Speed (m/s) : Inport  Port=2
  "2-D Lookup Table: T/T0 as f(Mach, Altitude)" : Lookup_n-D  BreakpointsForDimension1=linspace(0,0.6,52)  BreakpointsForDimension2=[0 5000 10000 15000]  Table=transpose(AircraftData.Propulsion.Interp.Thrust_Ratio_Interp_TO)  InternalRulePriority=Speed  RndMeth=Simplest
      settings: InputPortMap=u0,u1
  "2-D Lookup Table: TSFC as f(Mach, Altitude)" : Lookup_n-D  BreakpointsForDimension1=linspace(0,0.6,52)  BreakpointsForDimension2=[0 5000 10000 15000]  Table=transpose(AircraftData.Propulsion.tsfc2SI*AircraftData.Propulsion.Interp.TSFC_Interp_TO)  InternalRulePriority=Speed  RndMeth=Simplest
      settings: InputPortMap=u0,u1
  Divide : Product  Inputs=*/
  ISA Atmosphere Model : aerolibatmos2/ISA Atmosphere Model  useExtended=off  action=Warning  custom=off  viscosityOut=off  g=9.80665  gamma=1.4  R=287.0531  L=0.0065  h_trop=11000  h_strat=20000  rho0=1.225  P0=101325  T0=288.15  h0=0  S=110.4  Tref=273.15  muref=1.716e-5
  Ideal Airspeed Correction : aerolibasang/Ideal Airspeed Correction  units=Metric (MKS)  vel_in=TAS  vel_out_tas=CAS  vel_out_eas=TAS  vel_out_cas=TAS  method=Table Lookup  SubOnly=off  action=None
  Length Conversion : aerolibconvert2/Length Conversion  IU=m  OU=ft
  Max available thrust : Constant  Value=AircraftData.Propulsion.Thrust_0_TO
  Mux : Mux  Inputs=2
  Product : Product
  Scope : Scope  NumInputPorts=2
  Terminator : Terminator
  Max Thrust (N) : Outport
  TSFC kg/(N*s) : Outport  Port=2
  tag scope: Air_Density=global
  wires:
  Altitude (m)/1 -> Scope/2, Length Conversion/1, ISA Atmosphere Model/1
  ISA Atmosphere Model/2 -> Ideal Airspeed Correction/2, Divide/2
  Speed (m/s)/1 -> Mux/1, Ideal Airspeed Correction/1, Divide/1  "Airspeed (TAS, m/s)"
  Divide/1 -> "2-D Lookup Table: TSFC as f(Mach, Altitude)"/1, "2-D Lookup Table: T/T0 as f(Mach, Altitude)"/1  "Mach"
  Max available thrust/1 -> Product/1
  "2-D Lookup Table: T/T0 as f(Mach, Altitude)"/1 -> Product/2
  Product/1 -> Max Thrust (N)/1
  ISA Atmosphere Model/1 -> Terminator/1
  ISA Atmosphere Model/3 -> Ideal Airspeed Correction/3
  ISA Atmosphere Model/4 -> [Air_Density]
  Length Conversion/1 -> "2-D Lookup Table: TSFC as f(Mach, Altitude)"/2, "2-D Lookup Table: T/T0 as f(Mach, Altitude)"/2
  "2-D Lookup Table: TSFC as f(Mach, Altitude)"/1 -> TSFC kg/(N*s)/1
  Ideal Airspeed Correction/1 -> Mux/2  "Airspeed (CAS, m/s)"
  Mux/1 -> Scope/1

== system takeoff_13/A//C Reduced Order Dynamics/Triggered Subsystem1 ==
  time (s) : Inport
  Trigger : TriggerPort  VariantControl=(inherit)
  t_Hold_start : Outport
  wires:
  time (s)/1 -> t_Hold_start/1

== system takeoff_13/A//C Reduced Order Dynamics/Triggered Subsystem2 ==
  time (s) : Inport
  V (m/s) : Inport  Port=2
  s (m) : Inport  Port=3
  Trigger : TriggerPort  VariantControl=(inherit)
  t_LO : Outport
  V_LO : Outport  Port=2
  S_ground : Outport  Port=3
  wires:
  time (s)/1 -> t_LO/1
  V (m/s)/1 -> V_LO/1
  s (m)/1 -> S_ground/1

== system takeoff_13/AoA Control Law in climb/If t < t_ ==
  In1 : Inport
  Action Port : ActionPort  ActionPortLabel=else
  Out1 : Outport
  wires:
  In1/1 -> Out1/1

== system takeoff_13/AoA Control Law in climb/t > t_start_climb, t < t_start_level ==
  note: AoA Control Law
  gamma_c : Inport
  gamma : Inport  Port=2
  Action Port : ActionPort  ActionPortLabel=if(u1 > u2 & u1 < u3)
  PID Controller : slpidlib/PID Controller  Controller=PI  Form=Parallel  TimeDomain=Continuous-time  UseExternalTs=off  SampleTime=-1  IntegratorMethod=Forward Euler  FilterMethod=Forward Euler  ControllerParametersSource=internal  P=1.5  I=1  UseKiTs=off  D=1  UseExternalDerivativeSource=off  N=100  UseFilter=on  TunerSelectOption=Transfer Function Based (PID Tuner App)  InitialConditionSource=internal  InitialConditionForIntegrator=0  InitialConditionForFilter=0  DifferentiatorICPrevScaledInput=0  ExternalReset=none  TrackingMode=off  Kt=1  LimitOutput=off  SatLimitsSource=internal  UpperSaturationLimit=inf  LowerSaturationLimit=-inf  LinearizeAsGain=on  AntiWindupMode=none  Kb=1  LimitIntegrator=off  UpperIntegratorSaturationLimit=inf  LowerIntegratorSaturationLimit=-inf  POutMin=[]  POutMax=[]  IOutMin=[]  IOutMax=[]  DOutMin=[]  DOutMax=[]  NOutMin=[]  NOutMax=[]  SumOutMin=[]  SumOutMax=[]  SaturationOutMin=[]  SaturationOutMax=[]  PParamMin=[]  PParamMax=[]  IParamMin=[]  IParamMax=[]  DParamMin=[]  DParamMax=[]  NParamMin=[]  NParamMax=[]  KbParamMin=[]  KbParamMax=[]  KtParamMin=[]  KtParamMax=[]  KbOutMin=[]  KbOutMax=[]  KtOutMin=[]  KtOutMax=[]  IntegratorOutMin=[]  IntegratorOutMax=[]  FilterOutMin=[]  FilterOutMax=[]  SumI1OutMin=[]  SumI1OutMax=[]  SumI2OutMin=[]  SumI2OutMax=[]  SumI3OutMin=[]  SumI3OutMax=[]  SumI4OutMin=[]  SumI4OutMax=[]  SumDOutMin=[]  SumDOutMax=[]  DifferentiatorOutMin=[]  DifferentiatorOutMax=[]  FilterDiffOutCoefMin=[]  FilterDiffOutCoefMax=[]  ReciprocalOutMin=[]  ReciprocalOutMax=[]  SumDenOutMin=[]  SumDenOutMax=[]  SumNumOutMin=[]  SumNumOutMax=[]  DivideOutMin=[]  DivideOutMax=[]  UdiffTsProdOutMin=[]  UdiffTsProdOutMax=[]  NTsProdOutMin=[]  NTsProdOutMax=[]  UintegralTsProdOutMin=[]  UintegralTsProdOutMax=[]  UngainTsProdOutMin=[]  UngainTsProdOutMax=[]  ClampingZeroOutDataTypeStr=Inherit: Inherit via back propagation  ClampingZeroOutMin=[]  ClampingZeroOutMax=[]  FilterDenConstantOutDataTypeStr=Inherit: Inherit via back propagation  FilterDenConstantOutMin=[]  FilterDenConstantOutMax=[]  PCopyOutDataTypeStr=Inherit: Inherit via back propagation  PCopyOutMin=[]  PCopyOutMax=[]  NCopyOutDataTypeStr=Inherit: Inherit via back propagation  NCopyOutMin=[]  NCopyOutMax=[]  IntegratorContinuousStateAttributes=''  IntegratorStateMustResolveToSignalObject=off  IntegratorRTWStateStorageClass=Auto  FilterContinuousStateAttributes=''  FilterStateMustResolveToSignalObject=off  FilterRTWStateStorageClass=Auto  ParallelPVariant=InternalParameters  IdealPVariant=Disabled  IVariant=InternalParameters  DVariant=Disabled  IntegratorVariant=Continuous  SatVariant=Disabled  AWVariant=Passthrough  PCopyVariant=Disabled  TRVariant=Disabled  FdbkBlocksVariant=Forward  IdealPFdbkVariant=Disabled  SatFdbkVariant=Disabled  DerivativeFilterVariant=Disabled  NVariant=Disabled  NCopyVariant=Disabled_SignalSpec  FilterICVariant=Disabled  IntegratorICVariant=InternalICs  ExternalResetVariant=Disabled  TRSumVariant=Passthrough  SumFdbkVariant=Disabled  SumVariant=Sum_PI  TsampFilterVariant=InternalTs  TsampNgainVariant=Passthrough  TsampIntegralVariant=Disabled_SignalSpec  ExternalSaturationOutDataTypeStr=Inherit: Same as second input  DerivativeSourceVariant=Disabled  PreIntVariant=InternalPreInt
  Sum4 : Sum  Inputs=+-  InputSameDT=on  SaturateOnIntegerOverflow=on  OutDataTypeStr=Inherit: Same as first input
  Delta AoA : Outport  VectorParamsAs1DForOutWhenUnconnected=off
  wires:
  gamma_c/1 -> Sum4/1
  gamma/1 -> Sum4/2
  Sum4/1 -> PID Controller/1  "Error on gamma"
  PID Controller/1 -> Delta AoA/1  "AoA"

== system takeoff_13/AoA Control Law in climb/t > t_start_level ==
  note: AoA Control Law
  gamma_c : Inport
  gamma : Inport  Port=2
  Action Port : ActionPort  ActionPortLabel=elseif(u1 > u3)
  PID Controller : slpidlib/PID Controller  Controller=PI  Form=Parallel  TimeDomain=Continuous-time  UseExternalTs=off  SampleTime=-1  IntegratorMethod=Forward Euler  FilterMethod=Forward Euler  ControllerParametersSource=internal  P=1.5  I=1.0  UseKiTs=off  D=1  UseExternalDerivativeSource=off  N=100  UseFilter=on  TunerSelectOption=Transfer Function Based (PID Tuner App)  InitialConditionSource=internal  InitialConditionForIntegrator=0  InitialConditionForFilter=0  DifferentiatorICPrevScaledInput=0  ExternalReset=none  TrackingMode=off  Kt=1  LimitOutput=off  SatLimitsSource=internal  UpperSaturationLimit=inf  LowerSaturationLimit=-inf  LinearizeAsGain=on  AntiWindupMode=none  Kb=1  LimitIntegrator=off  UpperIntegratorSaturationLimit=inf  LowerIntegratorSaturationLimit=-inf  POutMin=[]  POutMax=[]  IOutMin=[]  IOutMax=[]  DOutMin=[]  DOutMax=[]  NOutMin=[]  NOutMax=[]  SumOutMin=[]  SumOutMax=[]  SaturationOutMin=[]  SaturationOutMax=[]  PParamMin=[]  PParamMax=[]  IParamMin=[]  IParamMax=[]  DParamMin=[]  DParamMax=[]  NParamMin=[]  NParamMax=[]  KbParamMin=[]  KbParamMax=[]  KtParamMin=[]  KtParamMax=[]  KbOutMin=[]  KbOutMax=[]  KtOutMin=[]  KtOutMax=[]  IntegratorOutMin=[]  IntegratorOutMax=[]  FilterOutMin=[]  FilterOutMax=[]  SumI1OutMin=[]  SumI1OutMax=[]  SumI2OutMin=[]  SumI2OutMax=[]  SumI3OutMin=[]  SumI3OutMax=[]  SumI4OutMin=[]  SumI4OutMax=[]  SumDOutMin=[]  SumDOutMax=[]  DifferentiatorOutMin=[]  DifferentiatorOutMax=[]  FilterDiffOutCoefMin=[]  FilterDiffOutCoefMax=[]  ReciprocalOutMin=[]  ReciprocalOutMax=[]  SumDenOutMin=[]  SumDenOutMax=[]  SumNumOutMin=[]  SumNumOutMax=[]  DivideOutMin=[]  DivideOutMax=[]  UdiffTsProdOutMin=[]  UdiffTsProdOutMax=[]  NTsProdOutMin=[]  NTsProdOutMax=[]  UintegralTsProdOutMin=[]  UintegralTsProdOutMax=[]  UngainTsProdOutMin=[]  UngainTsProdOutMax=[]  ClampingZeroOutDataTypeStr=Inherit: Inherit via back propagation  ClampingZeroOutMin=[]  ClampingZeroOutMax=[]  FilterDenConstantOutDataTypeStr=Inherit: Inherit via back propagation  FilterDenConstantOutMin=[]  FilterDenConstantOutMax=[]  PCopyOutDataTypeStr=Inherit: Inherit via back propagation  PCopyOutMin=[]  PCopyOutMax=[]  NCopyOutDataTypeStr=Inherit: Inherit via back propagation  NCopyOutMin=[]  NCopyOutMax=[]  IntegratorContinuousStateAttributes=''  IntegratorStateMustResolveToSignalObject=off  IntegratorRTWStateStorageClass=Auto  FilterContinuousStateAttributes=''  FilterStateMustResolveToSignalObject=off  FilterRTWStateStorageClass=Auto  ParallelPVariant=InternalParameters  IdealPVariant=Disabled  IVariant=InternalParameters  DVariant=Disabled  IntegratorVariant=Continuous  SatVariant=Disabled  AWVariant=Passthrough  PCopyVariant=Disabled  TRVariant=Disabled  FdbkBlocksVariant=Forward  IdealPFdbkVariant=Disabled  SatFdbkVariant=Disabled  DerivativeFilterVariant=Disabled  NVariant=Disabled  NCopyVariant=Disabled_SignalSpec  FilterICVariant=Disabled  IntegratorICVariant=InternalICs  ExternalResetVariant=Disabled  TRSumVariant=Passthrough  SumFdbkVariant=Disabled  SumVariant=Sum_PI  TsampFilterVariant=InternalTs  TsampNgainVariant=Passthrough  TsampIntegralVariant=Disabled_SignalSpec  ExternalSaturationOutDataTypeStr=Inherit: Same as second input  DerivativeSourceVariant=Disabled  PreIntVariant=InternalPreInt
  Sum4 : Sum  Inputs=+-  InputSameDT=on  SaturateOnIntegerOverflow=on  OutDataTypeStr=Inherit: Same as first input
  Delta AoA : Outport  VectorParamsAs1DForOutWhenUnconnected=off
  wires:
  gamma_c/1 -> Sum4/1
  gamma/1 -> Sum4/2
  Sum4/1 -> PID Controller/1  "Error on gamma"
  PID Controller/1 -> Delta AoA/1  "AoA"

== system takeoff_13/Commanded AoA/If t < t_Hold_start ==
  In1 : Inport
  Action Port : ActionPort  ActionPortLabel=else
  Out1 : Outport
  wires:
  In1/1 -> Out1/1

== system takeoff_13/Commanded AoA/If t <= t_Rot ==
  Action Port : ActionPort  ActionPortLabel=else
  zero : Constant  Value=0
  zero alpha_dot : Outport
  wires:
  zero/1 -> zero alpha_dot/1

== system takeoff_13/Commanded AoA/If t > t_Hold_start ==
  Action Port : ActionPort  ActionPortLabel=if(u1 > 0)
  zero : Constant  Value=0
  zero alpha_dot : Outport
  wires:
  zero/1 -> zero alpha_dot/1

== system takeoff_13/Commanded AoA/If t > t_Rot ==
  AoA (rad) : Inport
  Action Port : ActionPort  ActionPortLabel=if(u1 > 0)
  Add : Sum  Inputs=+-
  Constant : Constant
  Gain1 : Gain  Gain=alpha_dot_0
  Gain2 : Gain  Gain=k_alpha_Rot
  Cmd alpha_dot (rad/s) : Outport
  wires:
  Gain1/1 -> Cmd alpha_dot (rad/s)/1  "Cmd alpha_dot (rad/s)"
  AoA (rad)/1 -> Gain2/1
  Constant/1 -> Add/1
  Gain2/1 -> Add/2
  Add/1 -> Gain1/1

== system takeoff_13/Commanded AoA/Triggered Subsystem1 ==
  time (s) : Inport
  Trigger : TriggerPort  VariantControl=(inherit)
  t_Hold_start : Outport
  wires:
  time (s)/1 -> t_Hold_start/1

== system takeoff_13/Detect rotation time/Triggered Subsystem1 ==
  time (s) : Inport
  Trigger : TriggerPort  VariantControl=(inherit)
  t_rotation : Outport
  wires:
  time (s)/1 -> t_rotation/1

== system takeoff_13/Thrust Control Law/If t < t_ ==
  In1 : Inport
  Action Port : ActionPort  ActionPortLabel=else
  Out1 : Outport
  wires:
  In1/1 -> Out1/1

== system takeoff_13/Thrust Control Law/t > t_trim ==
  note: Thrust Control Law
  V_c : Inport
  V : Inport  Port=2
  Action Port : ActionPort  ActionPortLabel=if(u1 > u2 & u2 > 0)
  PID Controller : slpidlib/PID Controller  Controller=PI  Form=Parallel  TimeDomain=Continuous-time  UseExternalTs=off  SampleTime=-1  IntegratorMethod=Forward Euler  FilterMethod=Forward Euler  ControllerParametersSource=internal  P=1.8  I=2.5  UseKiTs=off  D=1  UseExternalDerivativeSource=off  N=100  UseFilter=on  TunerSelectOption=Transfer Function Based (PID Tuner App)  InitialConditionSource=internal  InitialConditionForIntegrator=0  InitialConditionForFilter=0  DifferentiatorICPrevScaledInput=0  ExternalReset=none  TrackingMode=off  Kt=1  LimitOutput=off  SatLimitsSource=internal  UpperSaturationLimit=inf  LowerSaturationLimit=-inf  LinearizeAsGain=on  AntiWindupMode=none  Kb=1  LimitIntegrator=off  UpperIntegratorSaturationLimit=inf  LowerIntegratorSaturationLimit=-inf  POutMin=[]  POutMax=[]  IOutMin=[]  IOutMax=[]  DOutMin=[]  DOutMax=[]  NOutMin=[]  NOutMax=[]  SumOutMin=[]  SumOutMax=[]  SaturationOutMin=[]  SaturationOutMax=[]  PParamMin=[]  PParamMax=[]  IParamMin=[]  IParamMax=[]  DParamMin=[]  DParamMax=[]  NParamMin=[]  NParamMax=[]  KbParamMin=[]  KbParamMax=[]  KtParamMin=[]  KtParamMax=[]  KbOutMin=[]  KbOutMax=[]  KtOutMin=[]  KtOutMax=[]  IntegratorOutMin=[]  IntegratorOutMax=[]  FilterOutMin=[]  FilterOutMax=[]  SumI1OutMin=[]  SumI1OutMax=[]  SumI2OutMin=[]  SumI2OutMax=[]  SumI3OutMin=[]  SumI3OutMax=[]  SumI4OutMin=[]  SumI4OutMax=[]  SumDOutMin=[]  SumDOutMax=[]  DifferentiatorOutMin=[]  DifferentiatorOutMax=[]  FilterDiffOutCoefMin=[]  FilterDiffOutCoefMax=[]  ReciprocalOutMin=[]  ReciprocalOutMax=[]  SumDenOutMin=[]  SumDenOutMax=[]  SumNumOutMin=[]  SumNumOutMax=[]  DivideOutMin=[]  DivideOutMax=[]  UdiffTsProdOutMin=[]  UdiffTsProdOutMax=[]  NTsProdOutMin=[]  NTsProdOutMax=[]  UintegralTsProdOutMin=[]  UintegralTsProdOutMax=[]  UngainTsProdOutMin=[]  UngainTsProdOutMax=[]  ClampingZeroOutDataTypeStr=Inherit: Inherit via back propagation  ClampingZeroOutMin=[]  ClampingZeroOutMax=[]  FilterDenConstantOutDataTypeStr=Inherit: Inherit via back propagation  FilterDenConstantOutMin=[]  FilterDenConstantOutMax=[]  PCopyOutDataTypeStr=Inherit: Inherit via back propagation  PCopyOutMin=[]  PCopyOutMax=[]  NCopyOutDataTypeStr=Inherit: Inherit via back propagation  NCopyOutMin=[]  NCopyOutMax=[]  IntegratorContinuousStateAttributes=''  IntegratorStateMustResolveToSignalObject=off  IntegratorRTWStateStorageClass=Auto  FilterContinuousStateAttributes=''  FilterStateMustResolveToSignalObject=off  FilterRTWStateStorageClass=Auto  ParallelPVariant=InternalParameters  IdealPVariant=Disabled  IVariant=InternalParameters  DVariant=Disabled  IntegratorVariant=Continuous  SatVariant=Disabled  AWVariant=Passthrough  PCopyVariant=Disabled  TRVariant=Disabled  FdbkBlocksVariant=Forward  IdealPFdbkVariant=Disabled  SatFdbkVariant=Disabled  DerivativeFilterVariant=Disabled  NVariant=Disabled  NCopyVariant=Disabled_SignalSpec  FilterICVariant=Disabled  IntegratorICVariant=InternalICs  ExternalResetVariant=Disabled  TRSumVariant=Passthrough  SumFdbkVariant=Disabled  SumVariant=Sum_PI  TsampFilterVariant=InternalTs  TsampNgainVariant=Passthrough  TsampIntegralVariant=Disabled_SignalSpec  ExternalSaturationOutDataTypeStr=Inherit: Same as second input  DerivativeSourceVariant=Disabled  PreIntVariant=InternalPreInt
  Sum4 : Sum  Inputs=+-  InputSameDT=on  SaturateOnIntegerOverflow=on  OutDataTypeStr=Inherit: Same as first input
  Delta delta_T : Outport  VectorParamsAs1DForOutWhenUnconnected=off
  wires:
  V_c/1 -> Sum4/1
  V/1 -> Sum4/2
  Sum4/1 -> PID Controller/1  "Error on V"
  PID Controller/1 -> Delta delta_T/1  "delta_T"
